simulink model "punto1"  (R2015a)
settings: Solver=ode45  StartTime=0.0  StopTime=20  RelTol=1e-3
settings Model: Creator=Administrador  LastModifiedBy=Administrador

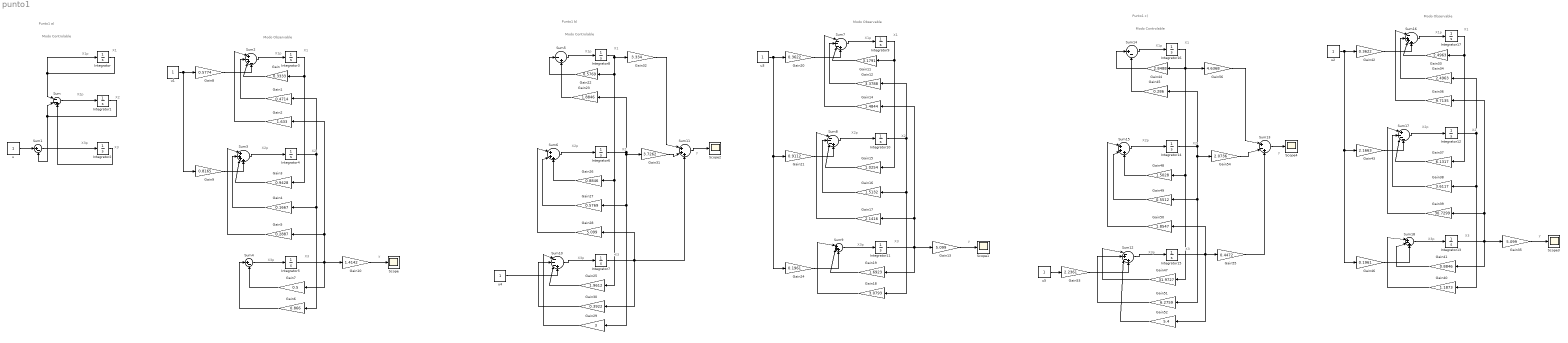
== system punto1 ==
  note: y
  note: X3
  note: X3p
  note: X1
  note: X1p
  note: X2p
  note: X2
  note: Punto1 a)
  note: Modo Observable
  note: Modo Controlable
  note: X3p
  note: X3
  note: X2
  note: X2p
  note: X1
  note: X1p
  note: y
  note: X3
  note: X3p
  note: X1
  note: X1p
  note: X2p
  note: X2
  note: Punto1 b)
  note: Modo Observable
  note: Modo Controlable
  note: y
  note: X3
  note: X3p
  note: X1
  note: X1p
  note: X2p
  note: X2
  note: y
  note: X3
  note: X3p
  note: X1
  note: X1p
  note: X2p
  note: X2
  note: Punto1 c)
  note: Modo Observable
  note: Modo Controlable
  note: y
  note: X3
  note: X3p
  note: X1
  note: X1p
  note: X2p
  note: X2
  Gain : Gain  Gain=0.3333
  Gain1 : Gain  Gain=0.4714
  Gain10 : Gain  Gain=1.4142
  Gain11 : Gain  Gain=3.1791
  Gain12 : Gain  Gain=3.3788
  Gain13 : Gain  Gain=5.099
  Gain14 : Gain  Gain=1.4844
  Gain15 : Gain  Gain=1.0254
  Gain16 : Gain  Gain=1.5132
  Gain17 : Gain  Gain=2.1416
  Gain18 : Gain  Gain=3.0793
  Gain19 : Gain  Gain=1.6923
  Gain2 : Gain  Gain=1.633
  Gain20 : Gain  Gain=0.3622
  Gain21 : Gain  Gain=0.9112
  Gain22 : Gain  Gain=0.5769
  Gain23 : Gain  Gain=1.8846
  Gain24 : Gain  Gain=0.1961
  Gain25 : Gain  Gain=1.9612
  Gain26 : Gain  Gain=0.8846
  Gain27 : Gain  Gain=0.5769
  Gain28 : Gain  Gain=5.099
  Gain29 : Gain  Gain=3
  Gain3 : Gain  Gain=0.9428
  Gain30 : Gain  Gain=0.3922
  Gain31 : Gain  Gain=3.7262
  Gain32 : Gain  Gain=3.334
  Gain33 : Gain  Gain=2.4963
  Gain34 : Gain  Gain=2.4963
  Gain35 : Gain  Gain=5.099
  Gain36 : Gain  Gain=9.7135
  Gain37 : Gain  Gain=6.1317
  Gain38 : Gain  Gain=3.6117
  Gain39 : Gain  Gain=30.7299
  Gain4 : Gain  Gain=0.1667
  Gain40 : Gain  Gain=1.1873
  Gain41 : Gain  Gain=0.8846
  Gain42 : Gain  Gain=0.3622
  Gain43 : Gain  Gain=2.1663
  Gain44 : Gain  Gain=2.8488
  Gain45 : Gain  Gain=0.286
  Gain46 : Gain  Gain=0.1961
  Gain47 : Gain  Gain=31.9727
  Gain48 : Gain  Gain=1.5028
  Gain49 : Gain  Gain=0.5512
  Gain5 : Gain  Gain=0.2887
  Gain50 : Gain  Gain=1.8547
  Gain51 : Gain  Gain=6.2759
  Gain52 : Gain  Gain=5.4
  Gain53 : Gain  Gain=2.2361
  Gain54 : Gain  Gain=2.0736
  Gain55 : Gain  Gain=0.4472
  Gain56 : Gain  Gain=4.6368
  Gain6 : Gain  Gain=0.866
  Gain7 : Gain  Gain=0.5
  Gain8 : Gain  Gain=0.5774
  Gain9 : Gain  Gain=0.8165
  Integrator{,1..17} (18 alike) : Integrator
  Scope{,1..4} (5 alike) : Scope
      Scope2 settings: SaveName=ScopeData2
      Scope3 settings: SaveName=ScopeData3
      Scope4 settings: SaveName=ScopeData4
  Sum : Sum  Inputs=|--+
  Sum1 : Sum  Inputs=|+-
  Sum10 : Sum  Inputs=|---+
  Sum{6,9,11,15} (4 alike) : Sum  Inputs=|+++
  Sum12 : Sum  Inputs=|-+-+
  Sum13 : Sum  Inputs=|+-+
  Sum14 : Sum  Inputs=|+-
  Sum16 : Sum  Inputs=|-+++
  Sum17 : Sum  Inputs=|+---
  Sum18 : Sum  Inputs=|+-+
  Sum2 : Sum  Inputs=|+-+-
  Sum3 : Sum  Inputs=|++++
  Sum4 : Sum  Inputs=|+-
  Sum5 : Sum  Inputs=|-+
  Sum7 : Sum  Inputs=|---+
  Sum8 : Sum  Inputs=|---+
  u{,1..5} (6 alike) : Constant
  wires:
  Integrator/1 -> Integrator/1, Sum/1
  Sum/1 -> Integrator1/1
  Integrator1/1 -> Sum/2, Sum1/2
  u/1 -> Sum1/1
  Integrator2/1 -> Sum/3
  Sum1/1 -> Integrator2/1
  Sum2/1 -> Integrator3/1
  Gain/1 -> Sum2/3
  Integrator3/1 -> Gain3/1, Gain/1
  Integrator4/1 -> Gain6/1, Gain4/1, Gain1/1
  Gain1/1 -> Sum2/2
  Integrator5/1 -> Gain10/1, Gain7/1, Gain2/1, Gain5/1
  Gain2/1 -> Sum2/1
  Sum3/1 -> Integrator4/1
  Gain3/1 -> Sum3/3
  Gain4/1 -> Sum3/2
  Gain5/1 -> Sum3/1
  Sum4/1 -> Integrator5/1
  Gain6/1 -> Sum4/1
  Gain7/1 -> Sum4/2
  u1/1 -> Gain9/1, Gain8/1
  Gain8/1 -> Sum2/4
  Gain9/1 -> Sum3/4
  Gain10/1 -> Scope/1
  Sum7/1 -> Integrator9/1
  Gain11/1 -> Sum7/3
  Integrator9/1 -> Gain15/1, Gain11/1
  Integrator10/1 -> Gain18/1, Gain16/1, Gain12/1
  Gain12/1 -> Sum7/2
  Integrator11/1 -> Gain13/1, Gain19/1, Gain14/1, Gain17/1
  Gain14/1 -> Sum7/1
  Sum8/1 -> Integrator10/1
  Gain15/1 -> Sum8/3
  Gain16/1 -> Sum8/2
  Gain17/1 -> Sum8/1
  Sum9/1 -> Integrator11/1
  Gain18/1 -> Sum9/1
  Gain19/1 -> Sum9/2
  u3/1 -> Gain24/1, Gain21/1, Gain20/1
  Gain20/1 -> Sum7/4
  Gain21/1 -> Sum8/4
  Gain13/1 -> Scope1/1
  Sum5/1 -> Integrator8/1
  Integrator6/1 -> Gain31/1, Gain29/1, Gain27/1, Gain23/1
  Sum6/1 -> Integrator6/1
  Gain26/1 -> Sum6/3
  Gain27/1 -> Sum6/2
  Gain28/1 -> Sum6/1
  Sum10/1 -> Integrator7/1
  Gain29/1 -> Sum10/1
  Gain30/1 -> Sum10/2
  Gain22/1 -> Sum5/1
  Gain23/1 -> Sum5/2
  Gain25/1 -> Sum10/3
  u4/1 -> Sum10/4
  Integrator8/1 -> Gain32/1, Gain25/1, Gain26/1, Gain22/1
  Gain31/1 -> Sum11/2
  Gain32/1 -> Sum11/1
  Integrator7/1 -> Sum11/3, Gain30/1, Gain28/1
  Sum11/1 -> Scope2/1
  Gain24/1 -> Sum9/3
  Sum16/1 -> Integrator17/1
  Gain33/1 -> Sum16/3
  Integrator17/1 -> Gain37/1, Gain33/1
  Integrator12/1 -> Gain40/1, Gain38/1, Gain34/1
  Gain34/1 -> Sum16/2
  Integrator13/1 -> Gain35/1, Gain41/1, Gain36/1, Gain39/1
  Gain36/1 -> Sum16/1
  Sum17/1 -> Integrator12/1
  Gain37/1 -> Sum17/3
  Gain38/1 -> Sum17/2
  Gain39/1 -> Sum17/1
  Sum18/1 -> Integrator13/1
  Gain40/1 -> Sum18/1
  Gain41/1 -> Sum18/2
  u2/1 -> Gain46/1, Gain43/1, Gain42/1
  Gain42/1 -> Sum16/4
  Gain43/1 -> Sum17/4
  Gain35/1 -> Scope3/1
  Sum14/1 -> Integrator16/1
  Integrator14/1 -> Gain54/1, Gain51/1, Gain49/1, Gain45/1
  Sum15/1 -> Integrator14/1
  Gain48/1 -> Sum15/3
  Gain49/1 -> Sum15/2
  Gain50/1 -> Sum15/1
  Sum12/1 -> Integrator15/1
  Gain44/1 -> Sum14/1
  Gain45/1 -> Sum14/2
  u5/1 -> Gain53/1
  Integrator16/1 -> Gain47/1, Gain48/1, Gain56/1, Gain44/1
  Integrator15/1 -> Gain55/1, Gain52/1, Gain50/1
  Gain46/1 -> Sum18/3
  Gain53/1 -> Sum12/4
  Gain47/1 -> Sum12/1
  Gain51/1 -> Sum12/2
  Gain52/1 -> Sum12/3
  Sum13/1 -> Scope4/1
  Gain54/1 -> Sum13/2
  Gain55/1 -> Sum13/3
  Gain56/1 -> Sum13/1
